simulink model "ej2"  (Simulink 8.5)
settings: Solver=ode3  StartTime=0  StopTime=2  FixedStep=1E-5  RelTol=1e-4
settings Model: Creator=dani  LastModifiedBy=dani
settings DataIOCC: LimitDataPoints=off  SignalLoggingSaveFormat=Dataset  Refine=10
settings OptimizationCC: ExpressionDepthLimit=128
settings DebuggingCC: UnderspecifiedInitializationDetection=Simplified  MergeDetectMultiDrivingBlocksExec=error  FcnCallInpInsideContextMsg=EnableAllAsError  StateNameClashWarn=none
settings GRTTargetCC: CombineOutputUpdateFcns=on  GRTInterface=off

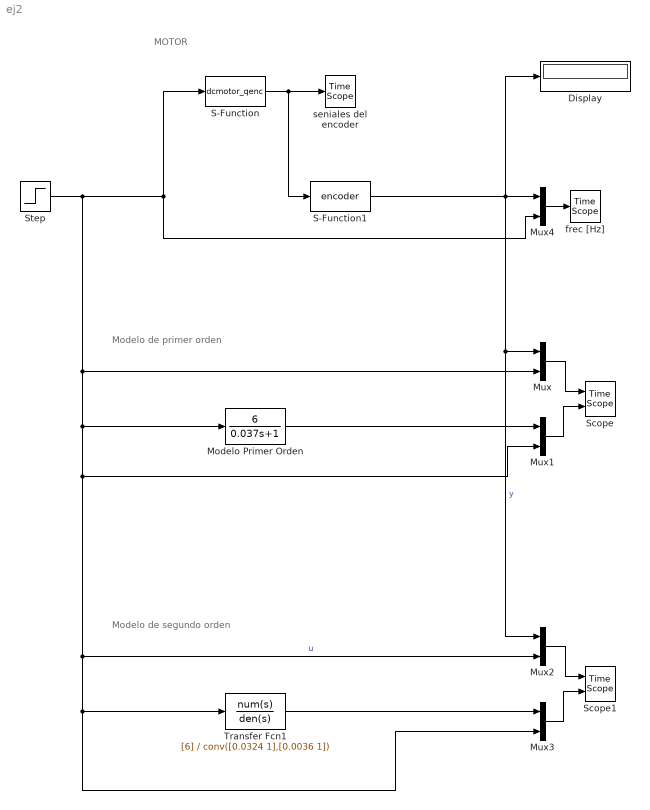
== system ej2 ==
  note: Modelo de primer orden
  note: MOTOR
  note: Modelo de segundo orden
  Display : Display
  Modelo Primer Orden : TransferFcn  Numerator=[6]  Denominator=[0.037 1]
  Mux{,1..4} (5 alike) : Mux  Inputs=2
  S-Function : S-Function  FunctionName=dcmotor_qenc  Parameters=10
  S-Function1 : S-Function  FunctionName=encoder  Parameters=1E-5 10
  Scope : TimeScope  NumInputPorts=2
  Scope1 : TimeScope  NumInputPorts=2
  Step : Step  After=12  SampleTime=0
  Transfer Fcn1 : TransferFcn  Numerator=[6]  Denominator=conv([0.0324 1],[0.0036 1])
  frec [Hz] : TimeScope
  seniales del encoder : TimeScope
  wires:
  S-Function/1 -> S-Function1/1, seniales del encoder/1
  Mux/1 -> Scope/1
  Modelo Primer Orden/1 -> Mux1/1
  Mux1/1 -> Scope/2
  Step/1 -> Modelo Primer Orden/1, Transfer Fcn1/1, Mux3/2, Mux2/2, Mux1/2, Mux/2, Mux4/2, S-Function/1  "u"
  S-Function1/1 -> Mux/1, Mux2/1, Mux4/1, Display/1  "y"
  Mux2/1 -> Scope1/1
  Transfer Fcn1/1 -> Mux3/1
  Mux3/1 -> Scope1/2
  Mux4/1 -> frec [Hz]/1
